simulink model "simul"  (R2020a)
settings: Solver=VariableStepAuto  StartTime=0.0  StopTime=10.0  RelTol=1e-3
libraries: simulink x2
settings Model: Creator=asus  LastModifiedBy=hirpej
settings DataIOCC: ReturnWorkspaceOutputs=off
settings OptimizationCC: LifeSpan=inf
settings DebuggingCC: SFExecutionAtInitializationDiag=none  ArithmeticOperatorsInVariantConditions=warning
settings SFSimCC: SimUseLocalCustomCode=off  CustomCodeUndefinedFunction=UseInterfaceOnly
settings RTWCC: RTWUseLocalCustomCode=off
settings CodeAppCC: StateflowObjectComments=on

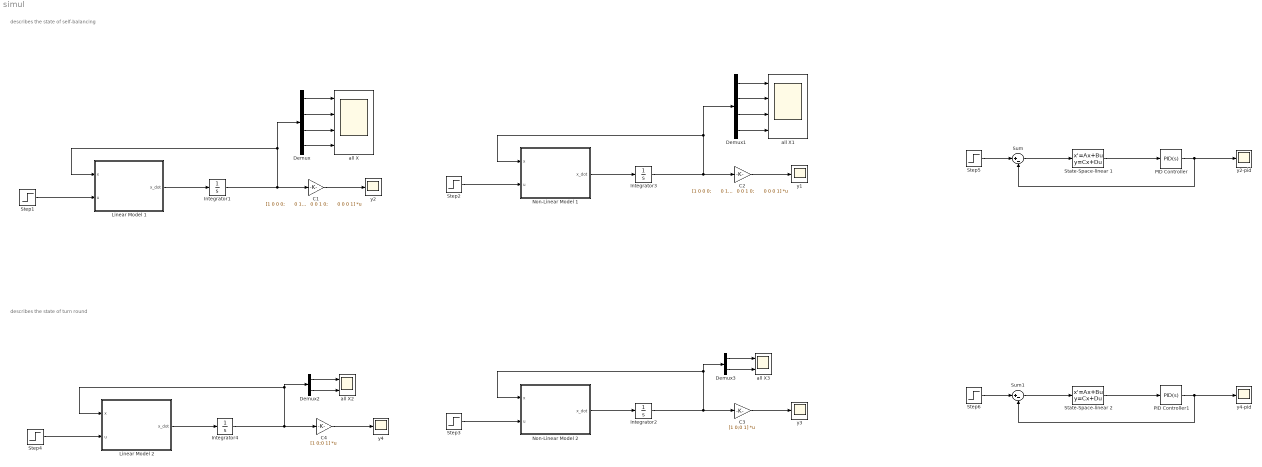
== system simul ==
  note: describes the state of self-balancing
  note: describes the state of turn round
  C1 : Gain  Gain=|  Multiplication=Matrix(K*u)
      | [1 0 0 0;
      |       0 1 0 0;
      |       0 0 1 0;
      |       0 0 0 1]
  C2 : Gain  Gain=|  Multiplication=Matrix(K*u)
      | [1 0 0 0;
      |       0 1 0 0;
      |       0 0 1 0;
      |       0 0 0 1]
  C3 : Gain  Gain=[1 0;0 1]  Multiplication=Matrix(K*u)
  C4 : Gain  Gain=[1 0;0 1]  Multiplication=Matrix(K*u)
  Demux : Demux
  Demux1 : Demux
  Demux2 : Demux  Outputs=2
  Demux3 : Demux  Outputs=2
  Integrator1 : Integrator  InitialCondition=[0 0 0 0]
  Integrator2 : Integrator  InitialCondition=[0 0]
  Integrator3 : Integrator  InitialCondition=[0 0 0 0]
  Integrator4 : Integrator  InitialCondition=[0 0]
  Linear Model 1 : MATLAB Function  TreatAsAtomicUnit=on
  Linear Model 2 : MATLAB Function  TreatAsAtomicUnit=on
  Non-Linear Model 1 : MATLAB Function  TreatAsAtomicUnit=on
  Non-Linear Model 2 : MATLAB Function  TreatAsAtomicUnit=on
  PID Controller : simulink/Continuous/PID Controller  Controller=PID  Form=Parallel  TimeDomain=Continuous-time  UseExternalTs=off  SampleTime=-1  IntegratorMethod=Forward Euler  FilterMethod=Forward Euler  ControllerParametersSource=internal  P=1.78631034235986  I=0  D=144.497917932766  UseFilter=on  N=53.8066590121805  TunerSelectOption=Transfer Function Based (PID Tuner App)  InitialConditionSource=internal  InitialConditionForIntegrator=0  InitialConditionForFilter=0  DifferentiatorICPrevScaledInput=0  ExternalReset=none  TrackingMode=off  Kt=1  LimitOutput=off  UpperSaturationLimit=inf  LowerSaturationLimit=-inf  LinearizeAsGain=on  AntiWindupMode=none  Kb=1  POutMin=[]  POutMax=[]  IOutMin=[]  IOutMax=[]  DOutMin=[]  DOutMax=[]  NOutMin=[]  NOutMax=[]  SumOutMin=[]  SumOutMax=[]  SaturationOutMin=[]  SaturationOutMax=[]  PParamMin=[]  PParamMax=[]  IParamMin=[]  IParamMax=[]  DParamMin=[]  DParamMax=[]  NParamMin=[]  NParamMax=[]  KbParamMin=[]  KbParamMax=[]  KtParamMin=[]  KtParamMax=[]  KbOutMin=[]  KbOutMax=[]  KtOutMin=[]  KtOutMax=[]  IntegratorOutMin=[]  IntegratorOutMax=[]  FilterOutMin=[]  FilterOutMax=[]  SumI1OutMin=[]  SumI1OutMax=[]  SumI2OutMin=[]  SumI2OutMax=[]  SumI3OutMin=[]  SumI3OutMax=[]  SumI4OutMin=[]  SumI4OutMax=[]  SumDOutMin=[]  SumDOutMax=[]  DifferentiatorOutMin=[]  DifferentiatorOutMax=[]  FilterDiffOutCoefMin=[]  FilterDiffOutCoefMax=[]  ReciprocalOutMin=[]  ReciprocalOutMax=[]  SumDenOutMin=[]  SumDenOutMax=[]  SumNumOutMin=[]  SumNumOutMax=[]  DivideOutMin=[]  DivideOutMax=[]  UdiffTsProdOutMin=[]  UdiffTsProdOutMax=[]  NTsProdOutMin=[]  NTsProdOutMax=[]  UintegralTsProdOutMin=[]  UintegralTsProdOutMax=[]  UngainTsProdOutMin=[]  UngainTsProdOutMax=[]  IntegratorContinuousStateAttributes=''  IntegratorStateMustResolveToSignalObject=off  IntegratorRTWStateStorageClass=Auto  FilterContinuousStateAttributes=''  FilterStateMustResolveToSignalObject=off  FilterRTWStateStorageClass=Auto  ParallelPVariant=InternalParameters  IdealPVariant=Disabled  IVariant=InternalParameters  DVariant=InternalParameters  IntegratorVariant=Continuous  SatVariant=Disabled  AWVariant=Passthrough  PCopyVariant=Disabled  TRVariant=Disabled  FdbkBlocksVariant=Forward  IdealPFdbkVariant=Disabled  SatFdbkVariant=Disabled  DerivativeFilterVariant=ContFilter  NVariant=InternalParameters  NCopyVariant=Disabled  FilterICVariant=InternalICsFilter  IntegratorICVariant=InternalICs  ExternalResetVariant=Disabled  TRSumVariant=Passthrough  SumFdbkVariant=Disabled  SumVariant=Sum_PID  TsampFilterVariant=InternalTs  TsampNgainVariant=Passthrough  TsampIntegralVariant=Passthrough
  PID Controller1 : simulink/Continuous/PID Controller  Controller=PID  Form=Parallel  TimeDomain=Continuous-time  UseExternalTs=off  SampleTime=-1  IntegratorMethod=Forward Euler  FilterMethod=Forward Euler  ControllerParametersSource=internal  P=0.43540556084688  I=0.102619675716169  D=0.383588183117973  UseFilter=on  N=14.518268107286  TunerSelectOption=Transfer Function Based (PID Tuner App)  InitialConditionSource=internal  InitialConditionForIntegrator=0  InitialConditionForFilter=0  DifferentiatorICPrevScaledInput=0  ExternalReset=none  TrackingMode=off  Kt=1  LimitOutput=off  UpperSaturationLimit=inf  LowerSaturationLimit=-inf  LinearizeAsGain=on  AntiWindupMode=none  Kb=1  POutMin=[]  POutMax=[]  IOutMin=[]  IOutMax=[]  DOutMin=[]  DOutMax=[]  NOutMin=[]  NOutMax=[]  SumOutMin=[]  SumOutMax=[]  SaturationOutMin=[]  SaturationOutMax=[]  PParamMin=[]  PParamMax=[]  IParamMin=[]  IParamMax=[]  DParamMin=[]  DParamMax=[]  NParamMin=[]  NParamMax=[]  KbParamMin=[]  KbParamMax=[]  KtParamMin=[]  KtParamMax=[]  KbOutMin=[]  KbOutMax=[]  KtOutMin=[]  KtOutMax=[]  IntegratorOutMin=[]  IntegratorOutMax=[]  FilterOutMin=[]  FilterOutMax=[]  SumI1OutMin=[]  SumI1OutMax=[]  SumI2OutMin=[]  SumI2OutMax=[]  SumI3OutMin=[]  SumI3OutMax=[]  SumI4OutMin=[]  SumI4OutMax=[]  SumDOutMin=[]  SumDOutMax=[]  DifferentiatorOutMin=[]  DifferentiatorOutMax=[]  FilterDiffOutCoefMin=[]  FilterDiffOutCoefMax=[]  ReciprocalOutMin=[]  ReciprocalOutMax=[]  SumDenOutMin=[]  SumDenOutMax=[]  SumNumOutMin=[]  SumNumOutMax=[]  DivideOutMin=[]  DivideOutMax=[]  UdiffTsProdOutMin=[]  UdiffTsProdOutMax=[]  NTsProdOutMin=[]  NTsProdOutMax=[]  UintegralTsProdOutMin=[]  UintegralTsProdOutMax=[]  UngainTsProdOutMin=[]  UngainTsProdOutMax=[]  IntegratorContinuousStateAttributes=''  IntegratorStateMustResolveToSignalObject=off  IntegratorRTWStateStorageClass=Auto  FilterContinuousStateAttributes=''  FilterStateMustResolveToSignalObject=off  FilterRTWStateStorageClass=Auto  ParallelPVariant=InternalParameters  IdealPVariant=Disabled  IVariant=InternalParameters  DVariant=InternalParameters  IntegratorVariant=Continuous  SatVariant=Disabled  AWVariant=Passthrough  PCopyVariant=Disabled  TRVariant=Disabled  FdbkBlocksVariant=Forward  IdealPFdbkVariant=Disabled  SatFdbkVariant=Disabled  DerivativeFilterVariant=ContFilter  NVariant=InternalParameters  NCopyVariant=Disabled  FilterICVariant=InternalICsFilter  IntegratorICVariant=InternalICs  ExternalResetVariant=Disabled  TRSumVariant=Passthrough  SumFdbkVariant=Disabled  SumVariant=Sum_PID  TsampFilterVariant=InternalTs  TsampNgainVariant=Passthrough  TsampIntegralVariant=Passthrough
  State-Space-linear 1 : StateSpace  A=|  B=|  C=[1 0 0 0]  D=0  InitialCondition=0
      A=|
      | [0 1 0 0;
      |      0  -15.0457 -1.0236 0;
      |      0 0 0 1;
      |      0 41.9119 0.1789 0]
      B=|
      | [0;
      |      0.1607;
      |       0;
      |       -0.3121]
  State-Space-linear 2 : StateSpace  A=|  B=|  C=[1 0 ]  D=0  InitialCondition=0
      A=|
      | [0 1;
      |       0 0]
      B=|
      | [0;
      |      9.782]
  Step{1..6} (6 alike) : Step  SampleTime=0
  Sum : Sum  Inputs=|+-
  Sum1 : Sum  Inputs=|+-
  all X : Scope  NumInputPorts=4
  all X1 : Scope  NumInputPorts=4
  all X2 : Scope  NumInputPorts=2
  all X3 : Scope  NumInputPorts=2
  y{1..4} (4 alike) : Scope
  y2-pid : Scope
  y4-pid : Scope
  wires:
  Step2/1 -> Non-Linear Model 1/2(u)
  Non-Linear Model 1/1(x_dot) -> Integrator3/1
  C2/1 -> y1/1
  Step3/1 -> Non-Linear Model 2/2(u)
  Non-Linear Model 2/1(x_dot) -> Integrator2/1
  C3/1 -> y3/1
  Step4/1 -> Linear Model 2/2(u)
  Linear Model 2/1(x_dot) -> Integrator4/1
  C4/1 -> y4/1
  Step1/1 -> Linear Model 1/2(u)
  Linear Model 1/1(x_dot) -> Integrator1/1
  C1/1 -> y2/1
  Integrator1/1 -> Demux/1, Linear Model 1/1(x), C1/1
  Demux/1 -> all X/1
  Demux/2 -> all X/2
  Demux/3 -> all X/3
  Demux/4 -> all X/4
  Integrator3/1 -> Demux1/1, Non-Linear Model 1/1(x), C2/1
  Demux1/1 -> all X1/1
  Demux1/2 -> all X1/2
  Demux1/3 -> all X1/3
  Demux1/4 -> all X1/4
  Integrator4/1 -> Demux2/1, Linear Model 2/1(x), C4/1
  Demux2/1 -> all X2/1
  Demux2/2 -> all X2/2
  Integrator2/1 -> Demux3/1, Non-Linear Model 2/1(x), C3/1
  Demux3/1 -> all X3/1
  Demux3/2 -> all X3/2
  Sum/1 -> State-Space-linear 1/1
  Step5/1 -> Sum/1
  State-Space-linear 1/1 -> PID Controller/1
  PID Controller/1 -> y2-pid/1, Sum/2
  Sum1/1 -> State-Space-linear 2/1
  Step6/1 -> Sum1/1
  PID Controller1/1 -> y4-pid/1, Sum1/2
  State-Space-linear 2/1 -> PID Controller1/1

== matlab function simul/Linear Model 2 ==
  data: x input; u input; x_dot output
function x_dot = fcn(x,u)

% system parameters
A2 = [0 1;
      0 0];
B2 = [0;
     9.782]; 
  
K2 =[ 16.7655    1.6357];
A2new  = A2-B2*K2;
  
x_dot= A2new * x + B2 * u;

== matlab function simul/Linear Model 1 ==
  data: x input; u input; x_dot output
function x_dot = fcn(x,u)

% system parameters
A1 = [0 1 0 0;
     0  -15.0457 -1.0236 0;
     0 0 0 1;
     0 41.9119 0.1789 0];
B1 = [0;
     0.1607;
      0;
      -0.3121];
  
K1 =[95.0239  -42.9217    2.7059    3.6789];
A1new  = A1-B1*K1;
  
x_dot= A1new * x + B1 * u;

== matlab function simul/Non-Linear Model 1 ==
  data: x input; u input; x_dot output
function x_dot = fcn(x,u)

% system parameters
M = 0.881; m = 0.015; R = 0.025; D = 0.137; L = 0.040;
Jw = 4.6875*10^(-6); Jp = 4.698667*10^(-4); g=9.8;
 
Kt = 0.02; Kb=0.02; Ra=1;
Kr = Kt/Ra;

A = [0.5*M*R+(m*R^2+Jw)/R , 0.5*R*L*M*cos(x(3)) , (D*(m*R^2+Jw))/(2*R);
     0.5*M*R+(m*R^2+Jw)/R , 0.5*R*L*M*cos(x(3)) , (-D*(m*R^2+Jw))/(2*R);
     2*L*M*cos(x(3)) , M*L^2*(cos(x(3)))^2 + Jp , 0];
 
B = [Kr*u-Kr*Kb*x(4)-0.5*R*L*M*x(4)^2*sin(x(3));
     Kr*u-Kr*Kb*x(4)-0.5*R*L*M*x(4)^2*sin(x(3));
   L*M*x(4)*sin(x(3))*x(2)+M*g*L*sin(x(3))+M*L^2*x(4)^2*sin(x(3))*cos(x(3))-Kr*u+Kr*Kb*x(4)];
 
M = inv(A) * B;


K1 =[95.0239  -42.9217    2.7059    3.6789];
u = K1*x ;

x_1_d=x(2);
x_2_d=M(1);
x_3_d=x(4);
x_4_d=M(2);

 


x_dot=[x_1_d;x_2_d;x_3_d;x_4_d];

== matlab function simul/Non-Linear Model 2 ==
  data: x input; u input; x_dot output
function x_dot = fcn(x,u)

% system parameters
A2 = [0 1;
      0 0];
B2 =  [0;
       259.5296];
  
K2 =[ 16.7655    1.6357];
A2new  = A2-B2*K2;
  
x_dot= A2new * x + B2 * u;
